simulink model "Test_Display"  (Simulink 8.1)
settings: Solver=ode45  SolverMode=SingleTasking  StartTime=0.0  StopTime=10.0  RelTol=1e-3
undefined symbols (not defined in the file): get, hot
libraries: dspsnks4 x1
(part 3 of 3)

== system Test_Display/Subsystem/Lamp ==

== system Test_Display/Subsystem/Lamp1 ==

== system Test_Display/Subsystem/Lamp10 ==

== system Test_Display/Subsystem/Lamp100 ==

== system Test_Display/Subsystem/Lamp101 ==

== system Test_Display/Subsystem/Lamp102 ==

== system Test_Display/Subsystem/Lamp103 ==

== system Test_Display/Subsystem/Lamp104 ==

== system Test_Display/Subsystem/Lamp105 ==

== system Test_Display/Subsystem/Lamp106 ==

== system Test_Display/Subsystem/Lamp107 ==

== system Test_Display/Subsystem/Lamp108 ==

== system Test_Display/Subsystem/Lamp109 ==

== system Test_Display/Subsystem/Lamp11 ==

== system Test_Display/Subsystem/Lamp110 ==

== system Test_Display/Subsystem/Lamp111 ==

== system Test_Display/Subsystem/Lamp112 ==

== system Test_Display/Subsystem/Lamp113 ==

== system Test_Display/Subsystem/Lamp114 ==

== system Test_Display/Subsystem/Lamp115 ==

== system Test_Display/Subsystem/Lamp116 ==

== system Test_Display/Subsystem/Lamp117 ==

== system Test_Display/Subsystem/Lamp118 ==

== system Test_Display/Subsystem/Lamp119 ==

== system Test_Display/Subsystem/Lamp12 ==

== system Test_Display/Subsystem/Lamp120 ==

== system Test_Display/Subsystem/Lamp121 ==

== system Test_Display/Subsystem/Lamp122 ==

== system Test_Display/Subsystem/Lamp123 ==

== system Test_Display/Subsystem/Lamp124 ==

== system Test_Display/Subsystem/Lamp125 ==

== system Test_Display/Subsystem/Lamp126 ==

== system Test_Display/Subsystem/Lamp127 ==

== system Test_Display/Subsystem/Lamp128 ==

== system Test_Display/Subsystem/Lamp129 ==

== system Test_Display/Subsystem/Lamp13 ==

== system Test_Display/Subsystem/Lamp130 ==

== system Test_Display/Subsystem/Lamp131 ==

== system Test_Display/Subsystem/Lamp132 ==

== system Test_Display/Subsystem/Lamp133 ==

== system Test_Display/Subsystem/Lamp134 ==

== system Test_Display/Subsystem/Lamp135 ==

== system Test_Display/Subsystem/Lamp136 ==

== system Test_Display/Subsystem/Lamp137 ==

== system Test_Display/Subsystem/Lamp138 ==

== system Test_Display/Subsystem/Lamp139 ==

== system Test_Display/Subsystem/Lamp14 ==

== system Test_Display/Subsystem/Lamp140 ==

== system Test_Display/Subsystem/Lamp141 ==

== system Test_Display/Subsystem/Lamp142 ==

== system Test_Display/Subsystem/Lamp143 ==

== system Test_Display/Subsystem/Lamp144 ==

== system Test_Display/Subsystem/Lamp145 ==

== system Test_Display/Subsystem/Lamp146 ==

== system Test_Display/Subsystem/Lamp147 ==

== system Test_Display/Subsystem/Lamp148 ==

== system Test_Display/Subsystem/Lamp149 ==

== system Test_Display/Subsystem/Lamp15 ==

== system Test_Display/Subsystem/Lamp150 ==

== system Test_Display/Subsystem/Lamp151 ==

== system Test_Display/Subsystem/Lamp152 ==

== system Test_Display/Subsystem/Lamp153 ==

== system Test_Display/Subsystem/Lamp154 ==

== system Test_Display/Subsystem/Lamp155 ==

== system Test_Display/Subsystem/Lamp156 ==

== system Test_Display/Subsystem/Lamp157 ==

== system Test_Display/Subsystem/Lamp158 ==

== system Test_Display/Subsystem/Lamp159 ==

== system Test_Display/Subsystem/Lamp16 ==

== system Test_Display/Subsystem/Lamp160 ==

== system Test_Display/Subsystem/Lamp161 ==

== system Test_Display/Subsystem/Lamp162 ==

== system Test_Display/Subsystem/Lamp163 ==

== system Test_Display/Subsystem/Lamp164 ==

== system Test_Display/Subsystem/Lamp165 ==

== system Test_Display/Subsystem/Lamp166 ==

== system Test_Display/Subsystem/Lamp167 ==

== system Test_Display/Subsystem/Lamp168 ==

== system Test_Display/Subsystem/Lamp169 ==

== system Test_Display/Subsystem/Lamp17 ==

== system Test_Display/Subsystem/Lamp170 ==

== system Test_Display/Subsystem/Lamp171 ==

== system Test_Display/Subsystem/Lamp172 ==

== system Test_Display/Subsystem/Lamp173 ==

== system Test_Display/Subsystem/Lamp174 ==

== system Test_Display/Subsystem/Lamp175 ==

== system Test_Display/Subsystem/Lamp176 ==

== system Test_Display/Subsystem/Lamp177 ==

== system Test_Display/Subsystem/Lamp178 ==

== system Test_Display/Subsystem/Lamp179 ==

== system Test_Display/Subsystem/Lamp18 ==

== system Test_Display/Subsystem/Lamp180 ==

== system Test_Display/Subsystem/Lamp181 ==

== system Test_Display/Subsystem/Lamp182 ==

== system Test_Display/Subsystem/Lamp183 ==

== system Test_Display/Subsystem/Lamp184 ==

== system Test_Display/Subsystem/Lamp185 ==

== system Test_Display/Subsystem/Lamp186 ==

== system Test_Display/Subsystem/Lamp187 ==

== system Test_Display/Subsystem/Lamp188 ==

== system Test_Display/Subsystem/Lamp189 ==

== system Test_Display/Subsystem/Lamp19 ==

== system Test_Display/Subsystem/Lamp190 ==

== system Test_Display/Subsystem/Lamp191 ==

== system Test_Display/Subsystem/Lamp192 ==

== system Test_Display/Subsystem/Lamp193 ==

== system Test_Display/Subsystem/Lamp194 ==

== system Test_Display/Subsystem/Lamp195 ==

== system Test_Display/Subsystem/Lamp196 ==

== system Test_Display/Subsystem/Lamp197 ==

== system Test_Display/Subsystem/Lamp198 ==

== system Test_Display/Subsystem/Lamp199 ==

== system Test_Display/Subsystem/Lamp2 ==

== system Test_Display/Subsystem/Lamp20 ==

== system Test_Display/Subsystem/Lamp200 ==

== system Test_Display/Subsystem/Lamp201 ==

== system Test_Display/Subsystem/Lamp202 ==

== system Test_Display/Subsystem/Lamp203 ==

== system Test_Display/Subsystem/Lamp204 ==

== system Test_Display/Subsystem/Lamp205 ==

== system Test_Display/Subsystem/Lamp206 ==

== system Test_Display/Subsystem/Lamp207 ==

== system Test_Display/Subsystem/Lamp208 ==

== system Test_Display/Subsystem/Lamp209 ==

== system Test_Display/Subsystem/Lamp21 ==

== system Test_Display/Subsystem/Lamp210 ==

== system Test_Display/Subsystem/Lamp211 ==

== system Test_Display/Subsystem/Lamp212 ==

== system Test_Display/Subsystem/Lamp213 ==

== system Test_Display/Subsystem/Lamp214 ==

== system Test_Display/Subsystem/Lamp215 ==

== system Test_Display/Subsystem/Lamp216 ==

== system Test_Display/Subsystem/Lamp217 ==

== system Test_Display/Subsystem/Lamp218 ==

== system Test_Display/Subsystem/Lamp219 ==

== system Test_Display/Subsystem/Lamp22 ==

== system Test_Display/Subsystem/Lamp220 ==

== system Test_Display/Subsystem/Lamp221 ==

== system Test_Display/Subsystem/Lamp222 ==

== system Test_Display/Subsystem/Lamp223 ==

== system Test_Display/Subsystem/Lamp224 ==

== system Test_Display/Subsystem/Lamp225 ==

== system Test_Display/Subsystem/Lamp226 ==

== system Test_Display/Subsystem/Lamp227 ==

== system Test_Display/Subsystem/Lamp228 ==

== system Test_Display/Subsystem/Lamp229 ==

== system Test_Display/Subsystem/Lamp23 ==

== system Test_Display/Subsystem/Lamp230 ==

== system Test_Display/Subsystem/Lamp231 ==

== system Test_Display/Subsystem/Lamp232 ==

== system Test_Display/Subsystem/Lamp233 ==

== system Test_Display/Subsystem/Lamp234 ==

== system Test_Display/Subsystem/Lamp235 ==

== system Test_Display/Subsystem/Lamp236 ==

== system Test_Display/Subsystem/Lamp237 ==

== system Test_Display/Subsystem/Lamp238 ==

== system Test_Display/Subsystem/Lamp239 ==

== system Test_Display/Subsystem/Lamp24 ==

== system Test_Display/Subsystem/Lamp240 ==

== system Test_Display/Subsystem/Lamp241 ==

== system Test_Display/Subsystem/Lamp242 ==

== system Test_Display/Subsystem/Lamp243 ==

== system Test_Display/Subsystem/Lamp244 ==

== system Test_Display/Subsystem/Lamp245 ==

== system Test_Display/Subsystem/Lamp246 ==

== system Test_Display/Subsystem/Lamp247 ==

== system Test_Display/Subsystem/Lamp248 ==

== system Test_Display/Subsystem/Lamp249 ==

== system Test_Display/Subsystem/Lamp25 ==

== system Test_Display/Subsystem/Lamp250 ==

== system Test_Display/Subsystem/Lamp251 ==

== system Test_Display/Subsystem/Lamp252 ==

== system Test_Display/Subsystem/Lamp253 ==

== system Test_Display/Subsystem/Lamp254 ==

== system Test_Display/Subsystem/Lamp255 ==

== system Test_Display/Subsystem/Lamp26 ==

== system Test_Display/Subsystem/Lamp27 ==

== system Test_Display/Subsystem/Lamp28 ==

== system Test_Display/Subsystem/Lamp29 ==

== system Test_Display/Subsystem/Lamp3 ==

== system Test_Display/Subsystem/Lamp30 ==

== system Test_Display/Subsystem/Lamp31 ==

== system Test_Display/Subsystem/Lamp32 ==

== system Test_Display/Subsystem/Lamp33 ==

== system Test_Display/Subsystem/Lamp34 ==

== system Test_Display/Subsystem/Lamp35 ==

== system Test_Display/Subsystem/Lamp36 ==

== system Test_Display/Subsystem/Lamp37 ==

== system Test_Display/Subsystem/Lamp38 ==

== system Test_Display/Subsystem/Lamp39 ==

== system Test_Display/Subsystem/Lamp4 ==

== system Test_Display/Subsystem/Lamp40 ==

== system Test_Display/Subsystem/Lamp41 ==

== system Test_Display/Subsystem/Lamp42 ==

== system Test_Display/Subsystem/Lamp43 ==

== system Test_Display/Subsystem/Lamp44 ==

== system Test_Display/Subsystem/Lamp45 ==

== system Test_Display/Subsystem/Lamp46 ==

== system Test_Display/Subsystem/Lamp47 ==

== system Test_Display/Subsystem/Lamp48 ==

== system Test_Display/Subsystem/Lamp49 ==

== system Test_Display/Subsystem/Lamp5 ==

== system Test_Display/Subsystem/Lamp50 ==

== system Test_Display/Subsystem/Lamp51 ==

== system Test_Display/Subsystem/Lamp52 ==

== system Test_Display/Subsystem/Lamp53 ==

== system Test_Display/Subsystem/Lamp54 ==

== system Test_Display/Subsystem/Lamp55 ==

== system Test_Display/Subsystem/Lamp56 ==

== system Test_Display/Subsystem/Lamp57 ==

== system Test_Display/Subsystem/Lamp58 ==

== system Test_Display/Subsystem/Lamp59 ==

== system Test_Display/Subsystem/Lamp6 ==

== system Test_Display/Subsystem/Lamp60 ==

== system Test_Display/Subsystem/Lamp61 ==

== system Test_Display/Subsystem/Lamp62 ==

== system Test_Display/Subsystem/Lamp63 ==

== system Test_Display/Subsystem/Lamp64 ==

== system Test_Display/Subsystem/Lamp65 ==

== system Test_Display/Subsystem/Lamp66 ==

== system Test_Display/Subsystem/Lamp67 ==

== system Test_Display/Subsystem/Lamp68 ==

== system Test_Display/Subsystem/Lamp69 ==

== system Test_Display/Subsystem/Lamp7 ==

== system Test_Display/Subsystem/Lamp70 ==

== system Test_Display/Subsystem/Lamp71 ==

== system Test_Display/Subsystem/Lamp72 ==

== system Test_Display/Subsystem/Lamp73 ==

== system Test_Display/Subsystem/Lamp74 ==

== system Test_Display/Subsystem/Lamp75 ==

== system Test_Display/Subsystem/Lamp76 ==

== system Test_Display/Subsystem/Lamp77 ==

== system Test_Display/Subsystem/Lamp78 ==

== system Test_Display/Subsystem/Lamp79 ==

== system Test_Display/Subsystem/Lamp8 ==

== system Test_Display/Subsystem/Lamp80 ==

== system Test_Display/Subsystem/Lamp81 ==

== system Test_Display/Subsystem/Lamp82 ==

== system Test_Display/Subsystem/Lamp83 ==

== system Test_Display/Subsystem/Lamp84 ==

== system Test_Display/Subsystem/Lamp85 ==

== system Test_Display/Subsystem/Lamp86 ==

== system Test_Display/Subsystem/Lamp87 ==

== system Test_Display/Subsystem/Lamp88 ==

== system Test_Display/Subsystem/Lamp89 ==

== system Test_Display/Subsystem/Lamp9 ==

== system Test_Display/Subsystem/Lamp90 ==

== system Test_Display/Subsystem/Lamp91 ==

== system Test_Display/Subsystem/Lamp92 ==

== system Test_Display/Subsystem/Lamp93 ==

== system Test_Display/Subsystem/Lamp94 ==

== system Test_Display/Subsystem/Lamp95 ==

== system Test_Display/Subsystem/Lamp96 ==

== system Test_Display/Subsystem/Lamp97 ==

== system Test_Display/Subsystem/Lamp98 ==
